simulink model "yori_command_window"  (R2023a)
settings: Solver=VariableStepAuto  StartTime=0.0  StopTime=10.0  RelTol=1e-3
model workspace (MAT data in the model file):
  Ts1 = 0.2
  Ts2 = 0.5
settings Model: Creator=HP  LastModifiedBy=HP

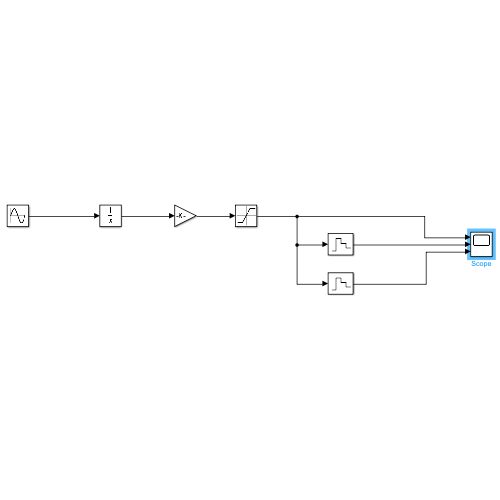
[thumbnail: Simulink's stored preview of the top-level diagram]
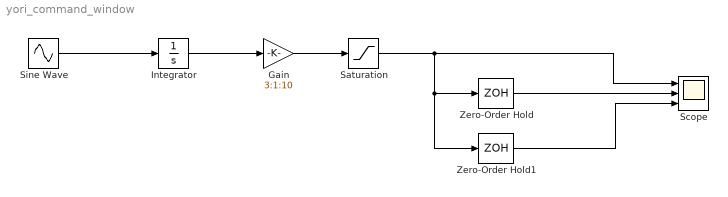
== system yori_command_window ==
  Gain : Gain  Gain=3:1:10
  Integrator : Integrator
  Saturation : Saturate  UpperLimit=rand(8,1)*10  LowerLimit=rand(8,1)*-10
  Scope : Scope  NumInputPorts=3
  Sine Wave : Sin  SampleTime=0
  Zero-Order Hold : ZeroOrderHold  SampleTime=Ts1
  Zero-Order Hold1 : ZeroOrderHold  SampleTime=Ts2
  wires:
  Gain/1 -> Saturation/1
  Integrator/1 -> Gain/1
  Sine Wave/1 -> Integrator/1
  Zero-Order Hold/1 -> Scope/2
  Saturation/1 -> Zero-Order Hold1/1, Zero-Order Hold/1, Scope/1
  Zero-Order Hold1/1 -> Scope/3
